simulink subsystem "IdealDCmotor_plant_model"  (R2024b)
settings: Solver=VariableStepAuto  StartTime=0.0  StopTime=10.0  RelTol=1e-3
libraries: cstblocks x1
settings Model: Creator=tshintai  LastModifiedBy=tshintai
settings SolverCC: AlgebraicLoopSolver=TrustRegion
settings OptimizationCC: ReuseModelBlockBuffer=off
settings DebuggingCC: UnconnectedInputMsg=warning  UnconnectedOutputMsg=warning  UnconnectedLineMsg=warning
settings ModelReferenceCC: EnableRefExpFcnMdlSchedulingChecks=on
settings RTWCC: GPUComputeCapability=3.5  DLArmComputeVersion=19.05

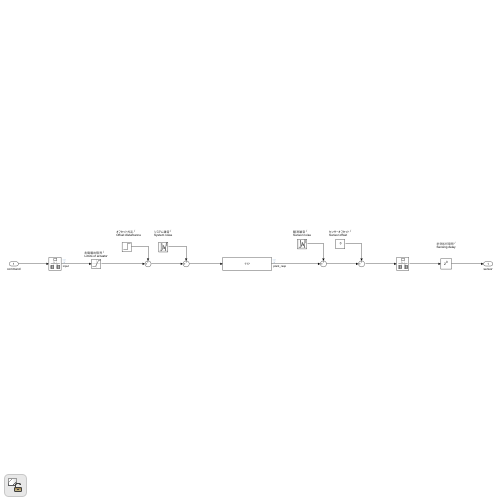
[thumbnail: Simulink's stored preview of the top-level diagram]
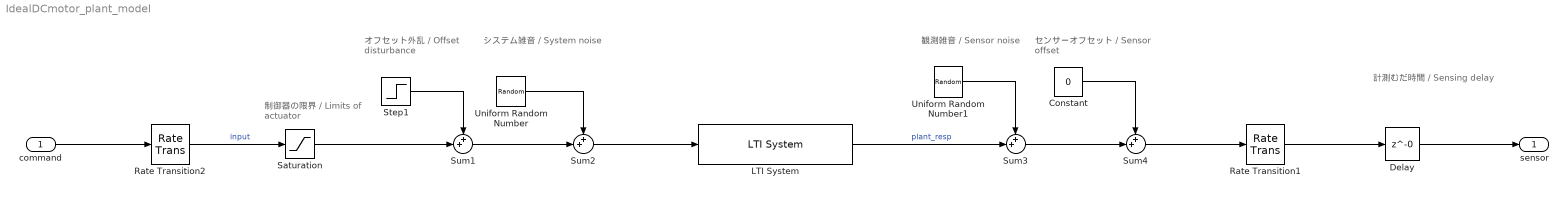
== system IdealDCmotor_plant_model ==
  note: オフセット外乱 /
      | Offset disturbance
  note: システム雑音 /
      | System noise
  note: 制御器の限界 /
      | Limits of actuator
  note: 計測むだ時間 /
      | Sensing delay
  note: センサーオフセット /
      | Sensor offset
  note: 観測雑音 /
      | Sensor noise
  command : Inport
  Constant : Constant  Value=0
  Delay : Delay  DelayLength=0
  LTI System : cstblocks/LTI System  sys=dc_motor_plant_sys  IC=[]  PadeOrder=0
  Rate Transition1 : RateTransition  OutPortSampleTime=TimeStep
  Rate Transition2 : RateTransition
  Saturation : Saturate  UpperLimit=220  LowerLimit=-220
  Step1 : Step  Time=5  After=0  SampleTime=0
  Sum{1..4} (4 alike) : Sum  Inputs=++|
  Uniform Random Number : UniformRandomNumber  Minimum=-0.2  Maximum=0.2  SampleTime=0
  Uniform Random Number1 : UniformRandomNumber  Minimum=-0.1  Maximum=0.1  Seed=1  SampleTime=0
  sensor : Outport
  wires:
  Uniform Random Number/1 -> Sum2/1
  Step1/1 -> Sum1/1
  Sum1/1 -> Sum2/2
  Rate Transition2/1 -> Saturation/1  "input"
  Saturation/1 -> Sum1/2
  Sum2/1 -> LTI System/1
  command/1 -> Rate Transition2/1
  Rate Transition1/1 -> Delay/1
  Sum4/1 -> Rate Transition1/1
  Delay/1 -> sensor/1
  Sum3/1 -> Sum4/2
  LTI System/1 -> Sum3/2  "plant_resp"
  Constant/1 -> Sum4/1
  Uniform Random Number1/1 -> Sum3/1
